simulink model "Fast_7DOF_eMPC_MC"  (R2024b)
settings: Solver=ode4  StartTime=0.0  StopTime=5  FixedStep=0.001  RelTol=1e-3
undefined symbols (not defined in the file): h_bump, Lb, M_vehicle, tau_act, v_vehicle, wheelbase
settings Model: Creator=THY  LastModifiedBy=THY

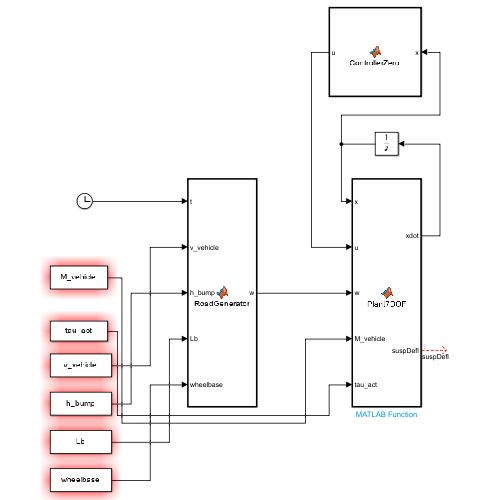
[thumbnail: Simulink's stored preview of the top-level diagram]
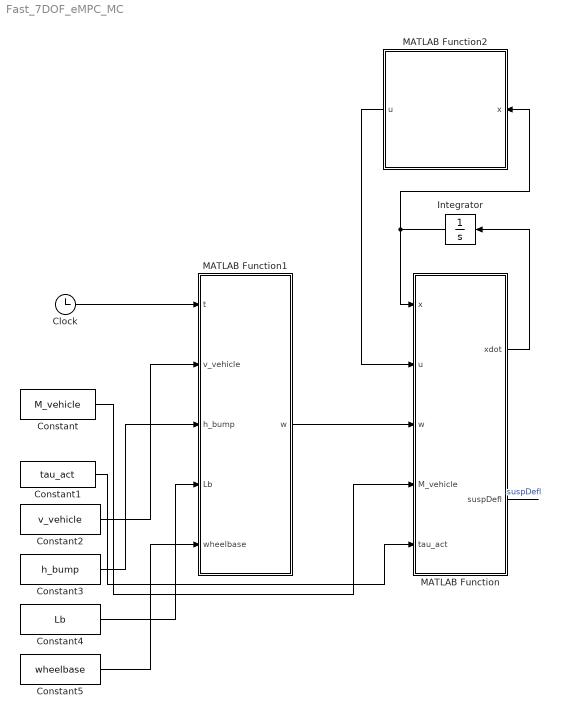
== system Fast_7DOF_eMPC_MC ==
  Clock : Clock
  Constant : Constant  Value=M_vehicle
  Constant1 : Constant  Value=tau_act
  Constant2 : Constant  Value=v_vehicle
  Constant3 : Constant  Value=h_bump
  Constant4 : Constant  Value=Lb
  Constant5 : Constant  Value=wheelbase
  Integrator : Integrator  InitialCondition=zeros(18,1)
  MATLAB Function : MATLAB Function  TreatAsAtomicUnit=on
  MATLAB Function1 : MATLAB Function  TreatAsAtomicUnit=on
  MATLAB Function2 : MATLAB Function  TreatAsAtomicUnit=on
  wires:
  MATLAB Function/1(xdot) -> Integrator/1
  Integrator/1 -> MATLAB Function2/1(x), MATLAB Function/1(x)
  MATLAB Function/2(suspDefl) -> ?  "suspDefl"
  MATLAB Function1/1(w) -> MATLAB Function/3(w)
  Clock/1 -> MATLAB Function1/1(t)
  MATLAB Function2/1(u) -> MATLAB Function/2(u)
  Constant2/1 -> MATLAB Function1/2(v_vehicle)
  Constant3/1 -> MATLAB Function1/3(h_bump)
  Constant4/1 -> MATLAB Function1/4(Lb)
  Constant5/1 -> MATLAB Function1/5(wheelbase)
  Constant/1 -> MATLAB Function/4(M_vehicle)
  Constant1/1 -> MATLAB Function/5(tau_act)

== matlab function Fast_7DOF_eMPC_MC/MATLAB Function1 ==
  data: t input; w output; v_vehicle input; h_bump input; Lb input; wheelbase input
function w = RoadGenerator(t, v_vehicle, h_bump, Lb, wheelbase)

t_delay = wheelbase / v_vehicle;

wFL = localBump(t,           v_vehicle, h_bump, Lb);
wFR = localBump(t,           v_vehicle, h_bump, Lb);
wRL = localBump(t - t_delay, v_vehicle, h_bump, Lb);
wRR = localBump(t - t_delay, v_vehicle, h_bump, Lb);

w = [wFL; wFR; wRL; wRR];

end

function y = localBump(t, v, h, Lb)

s = v * t;

if s >= 0 && s <= Lb
    y = 0.5*h*(1 - cos(2*pi*s/Lb));
else
    y = 0;
end

end

== matlab function Fast_7DOF_eMPC_MC/MATLAB Function ==
  data: x input; u input; xdot output; w input; M_vehicle input; tau_act input; suspDefl output
function [xdot, suspDefl] = Plant7DOF(x, u, w, M_vehicle, tau_act)
% 7DOF 垂向车辆模型 + 作动器一阶动力学
%
% x:
% [zs dzs theta dtheta phi dphi ...
%  zuFL dzuFL zuFR dzuFR zuRL dzuRL zuRR dzuRR ...
%  FaFL FaFR FaRL FaRR]'

% =========================
% 车辆参数：先用占位值，后续按你的车型修正
% =========================
M_nom = 2100;

muFL = 45;
muFR = 45;
muRL = 50;
muRR = 50;

mu = [muFL; muFR; muRL; muRR];

ms = M_vehicle - sum(mu);

% 转动惯量先按质量比例缩放
Ix_nom = 750;     % roll inertia [kg*m^2]，需要后续标定
Iy_nom = 2600;    % pitch inertia [kg*m^2]，需要后续标定

mass_scale = M_vehicle / M_nom;
Ix = Ix_nom * mass_scale;
Iy = Iy_nom * mass_scale;

% 轴距与轮距参数
lf = 1.25;        % CG 到前轴距离 [m]
lr = 1.55;        % CG 到后轴距离 [m]
tf = 1.60;        % 前轮距 [m]
tr = 1.60;        % 后轮距 [m]

% 悬架参数
ksFL = 30000;
ksFR = 30000;
ksRL = 35000;
ksRR = 35000;

csFL = 2500;
csFR = 2500;
csRL = 2500;
csRR = 2500;

ks = [ksFL; ksFR; ksRL; ksRR];
cs = [csFL; csFR; csRL; csRR];

% 轮胎刚度，先不考虑轮胎阻尼
ktFL = 230000;
ktFR = 230000;
ktRL = 250000;
ktRR = 250000;

kt = [ktFL; ktFR; ktRL; ktRR];

% 作动力饱和，和论文量级一致
uMax = 9000;
u = min(max(u(:), -uMax), uMax);

w = w(:);

% =========================
% 状态拆分
% =========================
zs     = x(1);
dzs    = x(2);
theta  = x(3);
dtheta = x(4);
phi    = x(5);
dphi   = x(6);

zu  = [x(7);  x(9);  x(11); x(13)];
dzu = [x(8);  x(10); x(12); x(14)];

Fa = [x(15); x(16); x(17); x(18)];

% =========================
% 车身四角位移
% 顺序：[FL FR RL RR]
% =========================
zb = [
    zs + lf*theta + tf/2*phi
    zs + lf*theta - tf/2*phi
    zs - lr*theta + tr/2*phi
    zs - lr*theta - tr/2*phi
];

dzb = [
    dzs + lf*dtheta + tf/2*dphi
    dzs + lf*dtheta - tf/2*dphi
    dzs - lr*dtheta + tr/2*dphi
    dzs - lr*dtheta - tr/2*dphi
];

% 悬架动挠度和速度
suspDefl = zb - zu;
dsusp = dzb - dzu;

% 作用在簧载质量上的四角力，向上为正
F_sprung = -ks .* suspDefl - cs .* dsusp + Fa;

% 簧载质量 heave / pitch / roll
ddzs = sum(F_sprung) / ms;

ddtheta = ( ...
    lf*(F_sprung(1) + F_sprung(2)) ...
  - lr*(F_sprung(3) + F_sprung(4)) ) / Iy;

ddphi = ( ...
    tf/2*(F_sprung(1) - F_sprung(2)) ...
  + tr/2*(F_sprung(3) - F_sprung(4)) ) / Ix;

% 非簧载质量动力学
% 对非簧载质量：悬架力反向，轮胎力为 -kt*(zu-w)
ddzu = zeros(4,1);

for i = 1:4
    F_unsprung = ks(i)*suspDefl(i) + cs(i)*dsusp(i) - Fa(i) ...
                 - kt(i)*(zu(i) - w(i));
    ddzu(i) = F_unsprung / mu(i);
end

% 作动器一阶动力学
dFa = (u - Fa) / tau_act;

% =========================
% 组装 xdot
% =========================
xdot = zeros(18,1);

xdot(1) = dzs;
xdot(2) = ddzs;

xdot(3) = dtheta;
xdot(4) = ddtheta;

xdot(5) = dphi;
xdot(6) = ddphi;

xdot(7)  = dzu(1);
xdot(8)  = ddzu(1);

xdot(9)  = dzu(2);
xdot(10) = ddzu(2);

xdot(11) = dzu(3);
xdot(12) = ddzu(3);

xdot(13) = dzu(4);
xdot(14) = ddzu(4);

xdot(15) = dFa(1);
xdot(16) = dFa(2);
xdot(17) = dFa(3);
xdot(18) = dFa(4);

end

== matlab function Fast_7DOF_eMPC_MC/MATLAB Function2 ==
  data: x input; u output
function u = ControllerZero(x)
% 第一阶段只验证 7DOF plant 和 Monte Carlo 框架
u = zeros(4,1);
end
